simulink model "full_sim"  (R2021b)
settings: Solver=FixedStepAuto  StartTime=0.0  StopTime=200  FixedStep=0.01  RelTol=1e-3
values from neighbouring files (symbols this model uses):
  F_g = 0.63    [lab3_workspace.m]
  J_ph = 0.04969    [lab3_workspace.m]
  J_ps = 1.1    [lab3_workspace.m]
  J_th = 1.1    [lab3_workspace.m]
  K_f = 0.0784    [lab3_workspace.m]
  K_ph_d = ((J_ph*(2*z_r*wn_r))/(K_f*l_h))*0.5    [lab3_workspace.m]
  K_ph_p = (J_ph*wn_r^2)/(K_f*l_h)    [lab3_workspace.m]
  K_r_i = 0.03*K_r_p    [lab3_workspace.m]
  K_r_p = (J_ps/(F_g*l_a*tau))*0.65    [lab3_workspace.m]
  K_th_d = ((J_th*(2*z_p*wn_p))/(K_f*l_a))    [lab3_workspace.m]
  K_th_i = 0.04*K_th_p    [lab3_workspace.m]
  K_th_p = ((J_th*wn_p^2)/(K_f*l_a))    [lab3_workspace.m]
  l_a = 0.63    [lab3_workspace.m]
  l_h = 0.18    [lab3_workspace.m]
settings Model: Creator=DSDLn  LastModifiedBy=DSDLn

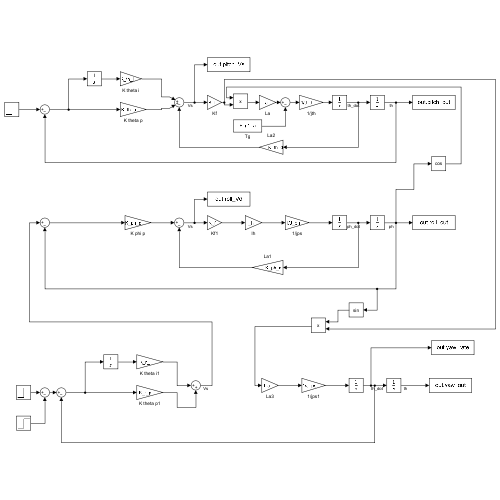
[thumbnail: Simulink's stored preview of the top-level diagram]
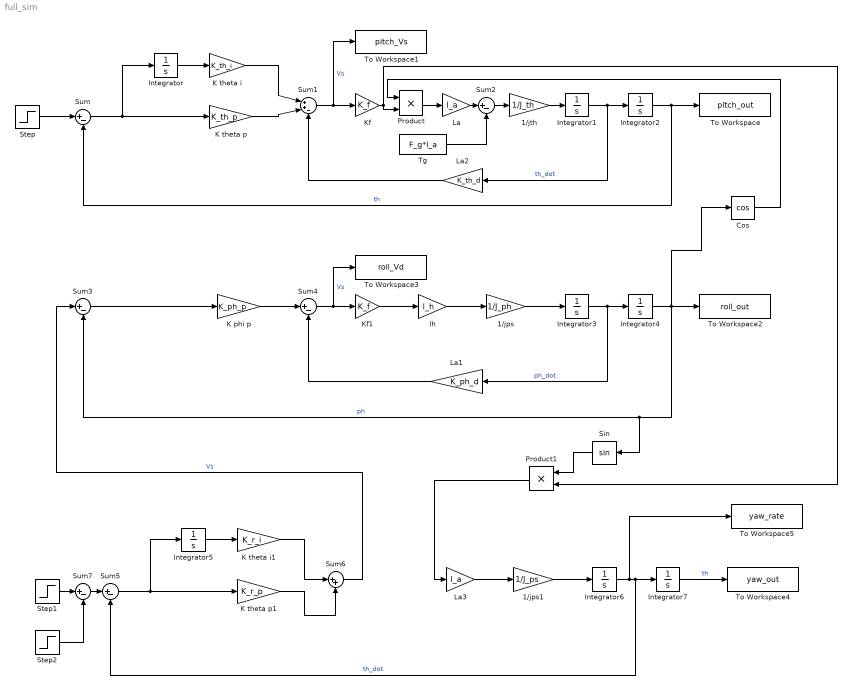
== system full_sim ==
  1/jps : Gain  Gain=1/J_ph
  1/jps1 : Gain  Gain=1/J_ps
  1/jth : Gain  Gain=1/J_th
  Cos : Trigonometry  Operator=cos
  Integrator{,1..7} (8 alike) : Integrator
  K phi p : Gain  Gain=K_ph_p
  K theta i : Gain  Gain=K_th_i
  K theta i1 : Gain  Gain=K_r_i
  K theta p : Gain  Gain=K_th_p
  K theta p1 : Gain  Gain=K_r_p
  Kf : Gain  Gain=K_f
  Kf1 : Gain  Gain=K_f
  La : Gain  Gain=l_a
  La1 : Gain  Gain=K_ph_d
  La2 : Gain  Gain=K_th_d
  La3 : Gain  Gain=l_a
  Product : Product
  Product1 : Product
  Sin : Trigonometry
  Step : Step  Time=100  After=deg2rad(20)  SampleTime=0.01
  Step1 : Step  Time=100  After=deg2rad(10)  SampleTime=0.01
  Step2 : Step  Time=118  After=deg2rad(10)  SampleTime=0.01
  Sum{,2..5,7} (6 alike) : Sum  Inputs=|+-
  Sum1 : Sum  Inputs=|++-
  Sum6 : Sum  Inputs=|++
  Tg : Constant  Value=F_g*l_a
  To Workspace : ToWorkspace  VariableName=pitch_out  SampleTime=-1
  To Workspace1 : ToWorkspace  VariableName=pitch_Vs  SampleTime=-1
  To Workspace2 : ToWorkspace  VariableName=roll_out  SampleTime=-1
  To Workspace3 : ToWorkspace  VariableName=roll_Vd  SampleTime=-1
  To Workspace4 : ToWorkspace  VariableName=yaw_out  SampleTime=-1
  To Workspace5 : ToWorkspace  VariableName=yaw_rate  SampleTime=-1
  lh : Gain  Gain=l_h
  wires:
  Step/1 -> Sum/1
  K theta p/1 -> Sum1/2
  Sum1/1 -> To Workspace1/1, Kf/1  "Vs"
  K theta i/1 -> Sum1/1
  1/jth/1 -> Integrator1/1
  Integrator1/1 -> Integrator2/1, La2/1  "th_dot"
  Integrator2/1 -> To Workspace/1, Sum/2  "th"
  Sum/1 -> K theta p/1, Integrator/1
  La2/1 -> Sum1/3
  Integrator/1 -> K theta i/1
  Product/1 -> La/1
  La/1 -> Sum2/1
  Sum2/1 -> 1/jth/1
  Tg/1 -> Sum2/2
  La1/1 -> Sum4/2
  Sum3/1 -> K phi p/1
  K phi p/1 -> Sum4/1
  Integrator3/1 -> Integrator4/1, La1/1  "ph_dot"
  1/jps/1 -> Integrator3/1
  lh/1 -> 1/jps/1
  Sum4/1 -> To Workspace3/1, Kf1/1  "Vs"
  Kf1/1 -> lh/1
  Integrator4/1 -> Sin/1, Sum3/2, Cos/1, To Workspace2/1  "ph"
  Cos/1 -> Product/1
  Step2/1 -> Sum7/2
  Step1/1 -> Sum7/1
  Integrator5/1 -> K theta i1/1
  Sum5/1 -> K theta p1/1, Integrator5/1
  Integrator7/1 -> To Workspace4/1  "th"
  Integrator6/1 -> Sum5/2, Integrator7/1, To Workspace5/1  "th_dot"
  La3/1 -> 1/jps1/1
  1/jps1/1 -> Integrator6/1
  K theta i1/1 -> Sum6/1
  K theta p1/1 -> Sum6/2
  Sum7/1 -> Sum5/1
  Sum6/1 -> Sum3/1  "Vs"
  Sin/1 -> Product1/1
  Kf/1 -> Product/2, Product1/2
  Product1/1 -> La3/1
